simulink model "db_pinon_cremallera"  (R2020a)
settings: Solver=VariableStepAuto  StartTime=0.0  StopTime=10  RelTol=1e-3
values from neighbouring files (symbols this model uses):
  B1 = 10    [pinon_cremallera.m]
  B2 = 50    [pinon_cremallera.m]
  J = 0.01    [motor_dc.m]    (also in pinon_cremallera.m = 0.1)
  K = 10    [pinon_cremallera.m]
  M = 100    [pinon_cremallera.m]
  R = 1e3    (= 1000)    [ejemplo_mallas_1.m]    (also in motor_dc.m = 10; pinon_cremallera.m = 0.01; sim_rlc.m)
settings Model: Creator=cmparedes  LastModifiedBy=cmparedes

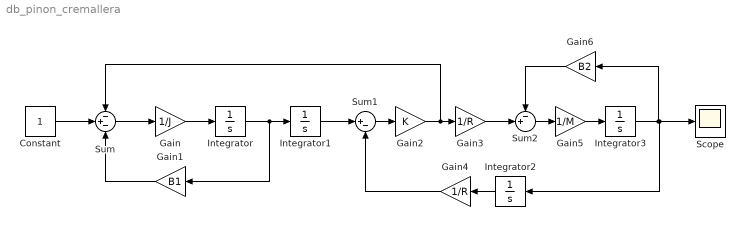
== system db_pinon_cremallera ==
  Constant : Constant
  Gain : Gain  Gain=1/J
  Gain1 : Gain  Gain=B1
  Gain2 : Gain  Gain=K
  Gain3 : Gain  Gain=1/R
  Gain4 : Gain  Gain=1/R
  Gain5 : Gain  Gain=1/M
  Gain6 : Gain  Gain=B2
  Integrator{,1..3} (4 alike) : Integrator
  Scope : Scope
  Sum : Sum  Inputs=-+-
  Sum1 : Sum  Inputs=|+-
  Sum2 : Sum  Inputs=-+|
  wires:
  Gain/1 -> Integrator/1
  Integrator/1 -> Integrator1/1, Gain1/1
  Integrator1/1 -> Sum1/1
  Sum1/1 -> Gain2/1
  Gain2/1 -> Sum/1, Gain3/1
  Gain4/1 -> Sum1/2
  Integrator2/1 -> Gain4/1
  Gain3/1 -> Sum2/2
  Sum2/1 -> Gain5/1
  Gain5/1 -> Integrator3/1
  Integrator3/1 -> Scope/1, Integrator2/1, Gain6/1
  Gain6/1 -> Sum2/1
  Gain1/1 -> Sum/3
  Sum/1 -> Gain/1
  Constant/1 -> Sum/2
